simulink model "晶闸管三相全控桥有源逆变"  (R2023a)
settings: Solver=VariableStepAuto  StartTime=0.0  StopTime=0.2  RelTol=1e-3
undefined symbols (not defined in the file): D1, lagging, pulse
libraries: spsThyristorLib x6, spsCurrentMeasurementLib x1, spsDCVoltageSourceLib x1, spsGroundLib x1, dspstat3 x1, spsPLLLib x1, spsPulseGeneratorThyristor6PulseLib x1, spsSeriesRLCBranchLib x1, spsThreePhaseVIMeasurementLib x1, spsThreePhaseSourceLib x1, spsVoltageMeasurementLib x1, spspowerguiLib x1
settings Model: Creator=17267  LastModifiedBy=17267

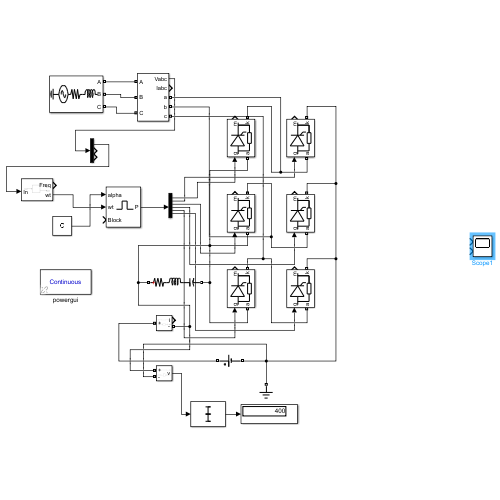
[thumbnail: Simulink's stored preview of the top-level diagram]
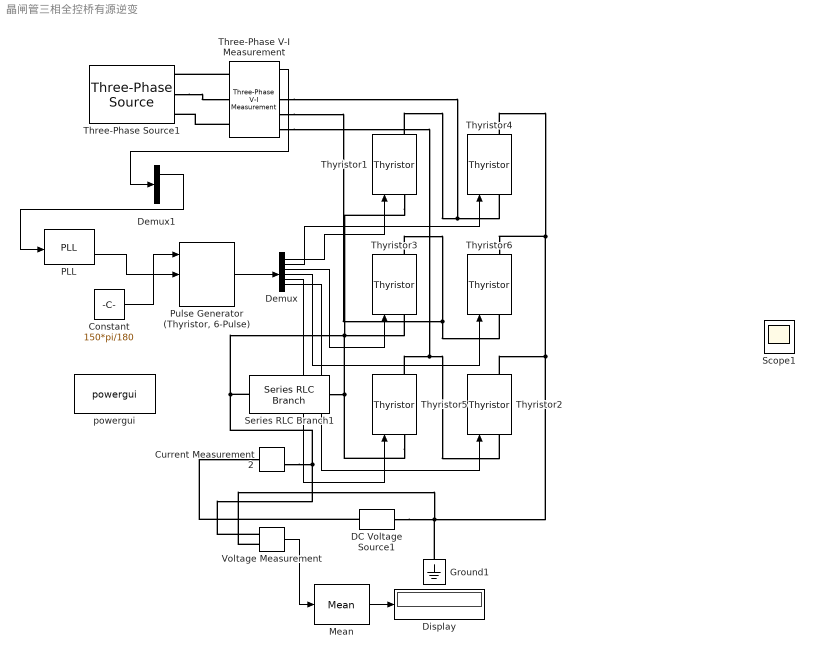
== system 晶闸管三相全控桥有源逆变 ==
  Constant : Constant  Value=150*pi/180
  Current Measurement2 : spsCurrentMeasurementLib/Current Measurement  PhasorSimulation=off  OutputType=Complex  PSBequivalent=0
  DC Voltage Source1 : spsDCVoltageSourceLib/DC Voltage Source  Amplitude=400  Measurements=None
  Demux : Demux  Outputs=6
  Demux1 : Demux  Outputs=3
  Display : Display
  Ground1 : spsGroundLib/Ground  LConnTagsString=a
  Mean : dspstat3/Mean  run=off  InputProcessing=Columns as channels (frame based)  reset_popup=None  directionMode=Each column  dimension=1  roiEnable=off  roiType=Rectangles  roiPortion=Entire ROI  roiOutput=Individual statistics for each ROI  roiFlag=off  roundingMode=Floor  overflowMode=off  outputDataTypeStr=Inherit: Same as accumulator  outputMin=[]  outputMax=[]  outputLastDataTypeStr=Inherit: Same as accumulator
  PLL : spsPLLLib/PLL  Fmin=50  Par_Init=[0, 50]  ParK=[180, 3200, 1]  TcD=1e-4  MaxRateChangeFreq=12  FilterCutOffFreq=25  Ts=0  AGC=on
      settings: LibrarySourceBlock=sps_lib/Control/PLL
  "Pulse Generator (Thyristor, 6-Pulse)" : spsPulseGeneratorThyristor6PulseLib/Pulse Generator (Thyristor, 6-Pulse)  GenType=6-pulse  Delta=D1 (lagging)  pwidth=60  Double_Pulse=off  Ts=0
      settings: LibrarySourceBlock=|
      | sps_lib/Power Electronics/Power Electronics Control/Pulse Generator
      | (Thyristor, 6-Pulse)
  Scope1 : Scope  NumInputPorts=2
  Series RLC Branch1 : spsSeriesRLCBranchLib/Series RLC Branch  LConnTagsString=__new0  RConnTagsString=__new0  BranchType=RLC  Resistance=0  Inductance=0.05  SetiL0=off  InitialCurrent=0  Capacitance=0  Setx0=off  InitialVoltage=0  Measurements=None
  Three-Phase V-I Measurement : spsThreePhaseVIMeasurementLib/Three-Phase V-I Measurement  VoltageMeasurement=phase-to-ground  SetLabelV=off  LabelV=Vabc  Vpu=off  VpuLL=off  CurrentMeasurement=yes  SetLabelI=off  LabelI=Iabc  Ipu=off  Pbase=100e6  Vbase=500e3  OutputType=Complex  PhasorSimulation=off  PSBequivalent=0
  Three-Phase Source1 : spsThreePhaseSourceLib/Three-Phase Source  InternalConnection=Yg  VoltagePhases=off  Voltage=381  PhaseAngle=0  Voltage_phases=[25e3 25e3 25e3]/sqrt(3)  PhaseAngles_phases=[0 -120 +120]  Frequency=50  NonIdealSource=on  SpecifyImpedance=off  Resistance=1  Inductance=5e-3  ShortCircuitLevel=100e6  BaseVoltage=25e3  XRratio=7  BusType=swing  Pref=10e3  Qref=0  Prefabc=[10e3, 10e3, 10e3]  Qrefabc=[0, 0, 0]  Qmin=-inf  Qmax=inf
  Thyristor{1..6} (6 alike) : spsThyristorLib/Thyristor  Ron=0.001  Lon=0  Vf=0.8  IC=0  Rs=500  Cs=250e-9  Measurements=on
  Voltage Measurement : spsVoltageMeasurementLib/Voltage Measurement  PhasorSimulation=off  OutputType=Complex  PSBequivalent=0
  powergui : spspowerguiLib/powergui  Priority=1  SimulationMode=Continuous  SampleTime=50e-6  frequency=60  Iterations=50  frequencyindice=50  Pbase=100e6  ErrMax=1e-4  UnitsV=kV  UnitsW=MW  buscounter=0  FunctionMessages=off  echomessages=off  EnableUseOfTLC=off  CurrentSourceSwitches=off  DisableSnubberDevices=off  DisableRonSwitches=off  DisableVfSwitches=off  DisplayEquations=off  AutomaticDiscreteSolvers=off  SolverType=Tustin/Backward Euler (TBE)  Interpol=off  ExternalGateDelay=off  methode=off  Ts=100  x0status=blocks  SPID=on  SwTol=0  HookPort=off  NonlinearTolerance=1e-4  nMaxIteration=100  ContinueOnMaxIteration=off  RestoreLinks=warning  ResistiveCurrentMeasurement=off  Frange=[0:2:500]  Ylog=off  Xlog=on  ShowGrid=off  save=off  variable=ZData  structure=0  ZoomFFT=off  StartTime=0.0  cycles=1  DisplayStyle=1  fundamental=60  FreqAxis=off  MaxFrequency=1000  frequencyindicesteady=1  RmsSteady=1  display=off
  wires:
  Constant/1 -> "Pulse Generator (Thyristor, 6-Pulse)"/1
  PLL/2 -> "Pulse Generator (Thyristor, 6-Pulse)"/2
  Demux/1 -> Thyristor1/1
  Demux/2 -> Thyristor4/1
  Demux/3 -> Thyristor3/1
  Demux/4 -> Thyristor6/1
  Demux/5 -> Thyristor5/1
  Demux/6 -> Thyristor2/1
  "Pulse Generator (Thyristor, 6-Pulse)"/1 -> Demux/1
  Three-Phase V-I Measurement/1 -> Demux1/1
  Demux1/1 -> PLL/1
  Mean/1 -> Display/1
  Voltage Measurement/1 -> Mean/1
  connections:
  Thyristor1/RConn1 -- Three-Phase V-I Measurement/RConn1 -- Thyristor4/LConn1
  Thyristor3/RConn1 -- Three-Phase V-I Measurement/RConn2 -- Thyristor6/LConn1
  Thyristor5/RConn1 -- Thyristor2/LConn1 -- Three-Phase V-I Measurement/RConn3
  Thyristor5/LConn1 -- Voltage Measurement/LConn1 -- Current Measurement2/RConn1 -- Series RLC Branch1/LConn1 -- Thyristor1/LConn1 -- Thyristor3/LConn1 -- Series RLC Branch1/RConn1
  Thyristor4/RConn1 -- Ground1/LConn1 -- Voltage Measurement/LConn2 -- DC Voltage Source1/LConn1 -- Thyristor2/RConn1 -- Thyristor6/RConn1
  Three-Phase V-I Measurement/LConn1 -- Three-Phase Source1/RConn1
  Three-Phase Source1/RConn2 -- Three-Phase V-I Measurement/LConn2
  Three-Phase V-I Measurement/LConn3 -- Three-Phase Source1/RConn3
  DC Voltage Source1/RConn1 -- Current Measurement2/LConn1
